simulink library "Library_Betriebsstrategie"  (R2018b)
settings: Solver=VariableStepAuto  StartTime=0.0  StopTime=10.0  RelTol=1e-3  EnableMultiTasking=on
undefined symbols (not defined in the file): akt_eUELG_HA, akt_eUELG_VA, akt_keinMVS_HA, akt_keinMVS_VA, akt_LSD_HA, akt_LSD_VA, akt_mUELG_HA, akt_mUELG_VA, akt_OD_HA, akt_OD_VA, DiscIntNeverNeededParam, magnitude, mu_road, mu_road_LF, mu_road_LR, mu_road_RF, mu_road_RR, par_MDT, par_VEH, stepsize
libraries: simulink x13
(part 6 of 6)

== matlab function Library_Betriebsstrategie/Momentverteilung_LR2/Radmomentenaufteilung/Optimierung rechts/Optimierung rechts ==
  data: M_wheel_right input; omega_RF input; omega_RR input; eta_RF input; eta_RR input; C output; D output; E output; v_slip_RF input; v_slip_RR input; gammaR output; min_P_loss output; Fz_RF input; Fz_RR input; Fy_RF input; Fy_RR input; r input
function [C, D, E, gammaR, min_P_loss] = fcn(M_wheel_right, omega_RF, omega_RR, eta_RF, eta_RR, v_slip_RF, v_slip_RR, Fz_RF, Fz_RR, Fy_RF, Fy_RR, r)

%% Diskrete Variable x (1 Prozent Schritte für Radmomentverteilung) und Initialisierung
step = 0.01;
x = [0:step:1];
n = 1/step + 1;
Einser = ones(1,n);
K_loss = 1;
K_slip = 1;
K_traction = 10;

%% Leistungsverluste in Abhängigkeit vom Antreiben oder Rekuperieren
if M_wheel_right >= 0 %vorne
    P_loss_f = ((Einser ./ eta_RF - 1)*omega_RF*M_wheel_right) .* x;
else
    P_loss_f = ((1 - eta_RF)*omega_RF*M_wheel_right) .* x;
end

if M_wheel_right >= 0 %hinten
    P_loss_r = ((Einser ./ eta_RR - 1)*omega_RR*M_wheel_right) .* (1-x);
else
    P_loss_r = ((1 - eta_RR)*omega_RR*M_wheel_right) .* (1-x);
end

%% Leistungsverluste in Abhängigkeit des Radschlupfes (also wird Traktion auch mit berücksichtigt)
P_slip_f = 5* abs(v_slip_RF * M_wheel_right/r) .* x;

P_slip_r = 5* abs(v_slip_RR * M_wheel_right/r) .* (1-x);

%% Ausnutzung des Kraftführungspotentials
mueT_RF = ((((M_wheel_right/r).*x).^2 + Fy_RF^2) ./ Fz_RF).^0.5;
mueT_RR = ((((M_wheel_right/r).*(1-x)).^2 + Fy_RR^2) ./ Fz_RR).^0.5;

%% Minimum der diskreten Leistungsverluste
P_loss = K_loss*(P_loss_f + P_loss_r) + K_slip*(P_slip_f + P_slip_r) + K_traction*(mueT_RF + mueT_RR);
[A, B] = min(P_loss);

%% Wertezuweisung
gammaR = step*B - step;
min_P_loss = A;

%% Analyse der Gewichtung bzw der Anteile an der Minimierungsfunktion
P_slip_rechts = K_slip*(P_slip_f + P_slip_r);
P_loss_rechts = K_loss*(P_loss_f + P_loss_r);
P_traction_rechts = K_traction*(mueT_RF + mueT_RR);
[C] = min(P_slip_rechts);
[D] = min(P_loss_rechts);
[E] = min(P_traction_rechts);

== matlab function Library_Betriebsstrategie/Momentverteilung_LR2/Limitierungen gesamt (mit MVS Limits)/Subsystem/MATLAB Function ==
  data: L1 input; Delta_T_f output; L2 input; L3 input; L4 input; L5 input; a_f input; a_r input; Delta_T_r output
function [Delta_T_f, Delta_T_r]  = fcn(L1, L2, L3, L4, L5, a_f, a_r)

%% Initialisierung
Delta_T_f=0;
Delta_T_r=0;

%% Zuweisung der maximalen TV Momente anhand der Antriebsstrangtopologie
if a_f == 3
    Delta_T_f=L5;
elseif a_f == 4
    Delta_T_f=L1;
elseif a_f == 5;
    Delta_T_f=L2;
end

if a_r == 3
    Delta_T_r=L5;
elseif a_r == 4
    Delta_T_r=L1;
elseif a_r == 5;
    Delta_T_r=L2;
end

%% Nomenklatur der Aktuatoren a_r und a_f
    % 1 = nur Elektromaschinen an der Achse
    % 2 = Offenes Differential an der Achse
    % 3 = Limited Slip Differential an der Achse
    % 4 = Elektrisches Überlagerungsgetriebe an der Achse
    % 5 = Mechanisches Überlagerungsgetriebe an der Achse

== matlab function Library_Betriebsstrategie/Momentenverteilung_Lagrange1/Limitierungen gesamt (mit MVS Limits)/Aktuatoren und Delta TV/Zuweisung Aktuatoren ==
  data: A1 input; A2 input; A3 input; A4 input; A5 input; a_f output; a_r output; A6 input; A7 input; A8 input; A9 input; A10 input
function [a_f, a_r]  = fcn(A1, A2, A3, A4, A5, A6, A7, A8, A9, A10)

%% Initialisierung
a_f=1;
a_r=1;

%% Zuweisung der Aktuatoren
% vorne
if A1 == 1
    a_f = 2;
elseif A2 == 1
    a_f = 3;
elseif A3 == 1
    a_f = 5;
elseif A4 == 1
    a_f = 4;
elseif A5 == 1
    a_f = 1;
end

% hinten
if A6 == 1
    a_r = 2;
elseif A7 == 1
    a_r = 3;
elseif A8 == 1
    a_r = 5;
elseif A9 == 1
    a_r = 4;
elseif A10 == 1
    a_r = 1;
end

%% Nomenklatur der Aktuatoren a_r und a_f
    % 1 = nur Elektromaschinen an der Achse
    % 2 = Offenes Differential an der Achse
    % 3 = Limited Slip Differential an der Achse
    % 4 = Elektrisches Überlagerungsgetriebe an der Achse
    % 5 = Mechanisches Überlagerungsgetriebe an der Achse

== matlab function Library_Betriebsstrategie/Momentenverteilung_Lagrange1/Limitierungen gesamt (mit MVS Limits)/Aktuatoren und Delta TV/TV Moment pro Achse ==
  data: L1 input; Delta_T_f output; L2 input; L3 input; L4 input; L5 input; a_f input; a_r input; Delta_T_r output
function [Delta_T_f, Delta_T_r]  = fcn(L1, L2, L3, L4, L5, a_f, a_r)

%% Initialisierung
Delta_T_f=0;
Delta_T_r=0;

%% Zuweisung der maximalen TV Momente anhand der Antriebsstrangtopologie
if a_f == 3
    Delta_T_f=L5;
elseif a_f == 4
    Delta_T_f=L1;
elseif a_f == 5;
    Delta_T_f=L2;
end

if a_r == 3
    Delta_T_r=L5;
elseif a_r == 4
    Delta_T_r=L1;
elseif a_r == 5;
    Delta_T_r=L2;
end

%% Nomenklatur der Aktuatoren a_r und a_f
    % 1 = nur Elektromaschinen an der Achse
    % 2 = Offenes Differential an der Achse
    % 3 = Limited Slip Differential an der Achse
    % 4 = Elektrisches Überlagerungsgetriebe an der Achse
    % 5 = Mechanisches Überlagerungsgetriebe an der Achse

== matlab function Library_Betriebsstrategie/Momentenverteilung_Lagrange1/Limitierungen gesamt (mit MVS Limits)/Limits Zusammenführung ==
  data: FxlimRF input; FxlimLF input; FxlimRR input; Fx_LF_ub output; Fx_LF_lb output; Fx_RF_ub output; Fx_RF_lb output; Fx_LR_ub output; Fx_LR_lb output; Fx_RR_ub output; Fx_RR_lb output; FxlimLR input; M_RF_ub input; M_RF_lb input; M_LF_ub input; M_LF_lb input; M_RR_ub input; M_RR_lb input; M_LR_ub input; M_LR_lb input; M_F_lb input; M_F_ub input; M_R_lb input; M_R_ub input; DELTA_T_f input; DELTA_T_r input; a_f input; a_r input; r input
function [Fx_LF_ub, Fx_LF_lb, Fx_RF_ub, Fx_RF_lb, Fx_LR_ub, Fx_LR_lb, Fx_RR_ub, Fx_RR_lb] = fcn(FxlimRF, FxlimLF, FxlimRR, FxlimLR, M_RF_ub, M_RF_lb, M_LF_ub, M_LF_lb, M_RR_ub, M_RR_lb, M_LR_ub, M_LR_lb, M_F_lb, M_F_ub, M_R_lb, M_R_ub,DELTA_T_f, DELTA_T_r,a_f, a_r, r)

%% Initialisierung der Limitationen auf die Reifen-Limits
Fx_LF_ub = FxlimLF;
Fx_RF_ub = FxlimRF;
Fx_LF_lb = (-1*FxlimLF);
Fx_RF_lb = (-1*FxlimRF);

Fx_LR_ub = FxlimLR;
Fx_RR_ub = FxlimRR;
Fx_LR_lb = (-1*FxlimLR);
Fx_RR_lb = (-1*FxlimRR);
    
%% Nomenklatur der Aktuatoren a_r und a_f
    % 1 = nur Elektromaschinen an der Achse
    % 2 = Offenes Differential an der Achse
    % 3 = Limited Slip Differential an der Achse
    % 4 = Elektrisches Überlagerungsgetriebe an der Achse
    % 5 = Mechanisches Überlagerungsgetriebe an der Achse
 
    
%% Nur Elektromotoren: Limit ist Minimum/Maximum aus Reifenlimit und Limit der EM
if a_f == 1
    Fx_LF_ub = min(FxlimLF,(M_LF_ub/r));
    Fx_RF_ub = min(FxlimRF,(M_RF_ub/r));
    Fx_LF_lb = max((-1*FxlimLF),(M_LF_lb/r));
    Fx_RF_lb = max((-1*FxlimRF),(M_RF_lb/r));
end

if a_r == 1
    Fx_LR_ub = min(FxlimLR,(M_LR_ub/r));
    Fx_RR_ub = min(FxlimRR,(M_RR_ub/r));
    Fx_LR_lb = max((-1*FxlimLR),(M_LR_lb/r));
    Fx_RR_lb = max((-1*FxlimRR),(M_RR_lb/r));
end

%% Offenes Differential: Limit ist Minimum/Maximum aus Reifenlimit und genau der Hälfte des max. Moments der achszentralen EM
if a_f == 2
    Fx_LF_ub = min(FxlimLF,(0.5*M_F_ub/r));
    Fx_RF_ub = min(FxlimRF,(0.5*M_F_ub/r));
    Fx_LF_lb = max((-1*FxlimLF),(0.5*M_F_lb/r));
    Fx_RF_lb = max((-1*FxlimRF),(0.5*M_F_lb/r));
end

if a_r == 2
    Fx_LR_ub = min(FxlimLR,(0.5*M_R_ub/r));
    Fx_RR_ub = min(FxlimRR,(0.5*M_R_ub/r));
    Fx_LR_lb = max((-1*FxlimLR),(0.5*M_R_lb/r));
    Fx_RR_lb = max((-1*FxlimRR),(0.5*M_R_lb/r));
end

%% Limited Slip Differential %% Elektrisches Überlagerungsgetriebe %% Mechanisches Überlagerungsgetriebe
if a_f >= 3 
    Fx_LF_ub = min(FxlimLF,(0.5*M_F_ub/r + 0.5*DELTA_T_f/r));
    Fx_RF_ub = min(FxlimRF,(0.5*M_F_ub/r + 0.5*DELTA_T_f/r));
    Fx_LF_lb = max((-1*FxlimLF),(0.5*M_F_lb/r - 0.5*DELTA_T_f/r));
    Fx_RF_lb = max((-1*FxlimRF),(0.5*M_F_lb/r - 0.5*DELTA_T_f/r));
end

if a_r >= 3
    Fx_LR_ub = min(FxlimLR,(0.5*M_R_ub/r + 0.5*DELTA_T_r/r));
    Fx_RR_ub = min(FxlimRR,(0.5*M_R_ub/r + 0.5*DELTA_T_r/r));
    Fx_LR_lb = max((-1*FxlimLR),(0.5*M_R_lb/r - 0.5*DELTA_T_r/r));
    Fx_RR_lb = max((-1*FxlimRR),(0.5*M_R_lb/r - 0.5*DELTA_T_r/r));
end

== matlab function Library_Betriebsstrategie/Momentenverteilung_Lagrange1/Radmomentenaufteilung/Limits berücksichtigen ==
  data: Fx_RF output; Fx_LF output; Fx_RR output; Fx_LF_ub input; Fx_LF_lb input; Fx_RF_ub input; Fx_RF_lb input; Fx_LR_ub input; Fx_LR_lb input; Fx_RR_ub input; Fx_RR_lb input; a_f input; a_r input; Fx_LR output; X_FL input; X_FR input; X_RL input; X_RR input
function [Fx_RF, Fx_LF, Fx_RR, Fx_LR] = fcn(Fx_LF_ub, Fx_LF_lb, Fx_RF_ub, Fx_RF_lb, Fx_LR_ub, Fx_LR_lb, Fx_RR_ub, Fx_RR_lb,a_f, a_r, X_FL, X_FR, X_RL, X_RR)

%% Initialisierung
Fx_RF = X_FR;
Fx_LF = X_FL;
Fx_RR = X_RR;
Fx_LR = X_RL;
    
%% Nomenklatur der Aktuatoren a_r und a_f
    % 1 = nur Elektromaschinen an der Achse
    % 2 = Offenes Differential an der Achse
    % 3 = Limited Slip Differential an der Achse
    % 4 = Elektrisches Überlagerungsgetriebe an der Achse
    % 5 = Mechanisches Überlagerungsgetriebe an der Achse
 
%% Algorithmus

    F_f= Fx_RF+Fx_LF;
    F_r= Fx_RR+Fx_LR;
  
  % Nur Elektromotoren:
  % Es werden radindividuell die Grenzen eingehalten. Die Differenzkräfte
  % werden zur späteren Verwendung gespeichert.
if a_f ==1
    if Fx_LF > Fx_LF_ub
        dFx_LF = Fx_LF-Fx_LF_ub;
        Fx_LF = Fx_LF_ub;
    end
    if Fx_RF > Fx_RF_ub
        dFx_RF = Fx_RF-Fx_RF_ub;
        Fx_RF = Fx_RF_ub;
    end
    if Fx_LF < Fx_LF_lb
        dFx_LF = Fx_LF-Fx_LF_lb;
        Fx_LF = Fx_LF_lb;
    end
    if Fx_RF < Fx_RF_lb
        dFx_RF = Fx_RF-Fx_RF_lb;
        Fx_RF = Fx_RF_lb;
    end
end

if a_r ==1
    if Fx_LR > Fx_LR_ub
        dFx_LR = Fx_LR-Fx_LR_ub;
        Fx_LR = Fx_LR_ub;
    end
    if Fx_RR > Fx_RR_ub
        dFx_RR = Fx_RR-Fx_RR_ub;
        Fx_RR = Fx_RR_ub;
    end
    if Fx_LR < Fx_LR_lb
        dFx_LR = Fx_LR-Fx_LR_lb;
        Fx_LR = Fx_LR_lb;
    end
    if Fx_RR < Fx_RR_lb
        dFx_RR = Fx_RR-Fx_RR_lb;
        Fx_RR = Fx_RR_lb;
    end
end

  % Offenes Differential:
  % ALSO keine TV Funktion der Achse.
  % Jedes Rad erhält die Hälfte der Gesamtachskraft.
  % Anschließend wird diese Kraft auf das Minimum der einzelnen Limits
  % gedeckelt.
  
if a_f ==2
    Fx_LF = F_f/2;
    Fx_RF = F_f/2;
    if Fx_LF > Fx_LF_ub || Fx_RF > Fx_RF_ub
        Fx_LF = min(Fx_LF_ub,Fx_RF_ub);
        Fx_RF = Fx_LF;
    end
    if Fx_LF < Fx_LF_lb || Fx_RF < Fx_RF_lb
        Fx_LF = max(Fx_LF_lb,Fx_RF_lb);
        Fx_RF = Fx_LF;
    end
end

if a_r ==2
    Fx_LR = F_r/2;
    Fx_RR = F_r/2;
    if Fx_LR > Fx_LR_ub || Fx_RR > Fx_RR_ub
        Fx_LR = min(Fx_LR_ub,Fx_RR_ub);
        Fx_RR = Fx_LR;
    end
    if Fx_LR < Fx_LR_lb || Fx_RR < Fx_RR_lb
        Fx_LR = max(Fx_LR_lb,Fx_RR_lb);
        Fx_RR = Fx_LR;
    end
end
    
%% Limited Slip Differential %% Elektrisches Überlagerungsgetriebe %% Mechanisches Überlagerungsgetriebe
if a_f >=3
    if Fx_LF > Fx_LF_ub
        dFx_LF = Fx_LF-Fx_LF_ub;
        Fx_LF = Fx_LF_ub;
    end
    if Fx_RF > Fx_RF_ub
        dFx_RF = Fx_RF-Fx_RF_ub;
        Fx_RF = Fx_RF_ub;
    end
    if Fx_LF < Fx_LF_lb
        dFx_LF = Fx_LF-Fx_LF_lb;
        Fx_LF = Fx_LF_lb;
    end
    if Fx_RF < Fx_RF_lb
        dFx_RF = Fx_RF-Fx_RF_lb;
        Fx_RF = Fx_RF_lb;
    end
end

if a_r >=3
    if Fx_LR > Fx_LR_ub
        dFx_LR = Fx_LR-Fx_LR_ub;
        Fx_LR = Fx_LR_ub;
    end
    if Fx_RR > Fx_RR_ub
        dFx_RR = Fx_RR-Fx_RR_ub;
        Fx_RR = Fx_RR_ub;
    end
    if Fx_LR < Fx_LR_lb
        dFx_LR = Fx_LR-Fx_LR_lb;
        Fx_LR = Fx_LR_lb;
    end
    if Fx_RR < Fx_RR_lb
        dFx_RR = Fx_RR-Fx_RR_lb;
        Fx_RR = Fx_RR_lb;
    end
end
    
%% Korrektur des TV Moments %% Korrektur des Gesamtmoments

== matlab function Library_Betriebsstrategie/Momentenverteilung_Lagrange1/Radmomentenaufteilung/Optimierung mit Lagrange Multiplikator Methode ==
  data: a_f input; a_r input; vslip_FL input; vslip_FR input; vslip_RL input; vslip_RR input; tF input; tR input; lf input; lr input; delta input; X_req input; Mz input; X_FL output; X_FR output; X_RL output; X_RR output; Z_FL input; Z_FR input; Z_RL input; Z_RR input; X_FL1 input; X_FR1 input; X_RL1 input; X_RR1 input
function [X_FL, X_FR, X_RL, X_RR] = fcn(a_f, a_r, vslip_FL, vslip_FR, vslip_RL, vslip_RR,tF, tR, lf, lr, delta, X_req, Mz, Z_FL, Z_FR, Z_RL, Z_RR, X_FL1, X_FR1, X_RL1, X_RR1)

%% Auswahl der Antriebsstrantopologie
a=1;
b=1;

if a_f ==2
    a=0;
end
if a_r ==2
    b=0;
end

if a_f ==2 && a_r==2
    a=1;
    b=1;
end

% TV vorne und hinten möglich a=1 und b=1
% TV nur vorne möglich a=1
% TV nur hinten möglich b=1
% kein TV möglich a=0 und b=0

%% Matrix für die Randbedingungen ( Gesamtmoment und TV Moment)
B0 = [cos(delta) cos(delta) 1 1; a*((-tF/2)*cos(delta)+lf*sin(delta)) a*((tF/2)*cos(delta)+lf*sin(delta)) b*(-tR/2) b*(tR/2)];
y0 = [X_req; Mz];

%% Algorithmus
    %% Initialbedingungen
i=0;    
B=B0;
y=y0;
     
    %% Verhindern abgehobener Räder
if Z_FL < 1
    Z_FL = 1;
    x_FL_max = 0;
end

if Z_FR < 1
    Z_FR = 1;
    x_FR_max = 0;
end

if Z_RL < 1
    Z_RL = 1;
    x_RL_max = 0;
end

if Z_RR < 1
    Z_RR = 1;
    x_RR_max = 0;
end

%% Matrizen für die Mimimierung
W1 = [1/Z_FL+abs(vslip_FL) 0 0 0; 0 1/Z_FR+abs(vslip_FR) 0 0; 0 0 1/Z_RL+abs(vslip_RL) 0; 0 0 0 1/Z_RR+abs(vslip_RR)];
W2 = 0.01 * eye(4);
Wquad = W1^2 + W2^2;
X_alt = [X_FL1; X_FR1; X_RL1; X_RR1];

%% Minimierungsargument
% min ||W1*x||^2 + ||W2*(x-x0)||^2
%   ||W1*x||^2 + ||W2*(x-x0)||^2 = xt*W1^2*x + (x-x0)t*W2^2*(x-x0)
%   = xt*(W1^2+W2^2)*x - 2*x*W2^2*x0 + x0*W2^2*x0
%   = xt*W^2*x - 2*x*W2^2*x0 + Konstante
%   mit W^2 = W1^2 + W2^2


%% Berechnung von Xij
G = (Wquad^(-1))*(B')*(B*(Wquad^(-1))*(B'))^(-1);
X = G*y + (eye(4)-G*B)*(Wquad^(-1))*(W2^2)*X_alt;


%% Ausgabewerte berechnen
X_FL = X(1);
X_FR = X(2);
X_RL = X(3);
X_RR = X(4);

%% Limits berücksichtigen
if a==0
    X_F = X_FL + X_FR;
    X_FL = X_F/2;
    X_FR = X_F/2;
end

if b==0
    X_R = X_RL + X_RR;
    X_RL = X_R/2;
    X_RR = X_R/2;
end

if a_f ==2 && a_r==2
    X_F = X_FL + X_FR;
    X_FL = X_F/2;
    X_FR = X_F/2;
    X_R = X_RL + X_RR;
    X_RL = X_R/2;
    X_RR = X_R/2;
end

== matlab function Library_Betriebsstrategie/Schaltstrategie/Schaltlogik ==
  data: delta_n_LF input; delta_n_RF input; delta_n_LR input; delta_n_RR input; delta_n_F input; delta_n_R input; delta_m_LF input; delta_m_RF input; delta_m_LR input; delta_m_RR input; delta_m_F input; delta_m_R input; idx_LF_eff input; idx_RF_eff input; idx_LR_eff input; idx_RR_eff input; idx_F_eff input; idx_R_eff input; i_LF output; i_RF output; i_LR output; i_RR output; i_F output; iv_LF input; iv_RF input; iv_LR input; iv_RR input; iv_F input; iv_R input; i_R output; idx_LF output; idx_RF output; idx_LR output; idx_RR output; idx_F output; idx_R output; idx_LF_alt input; idx_RF_alt input; idx_LR_alt input; idx_RR_alt input; idx_F_alt input; idx_R_alt input
function [i_LF, i_RF, i_LR, i_RR, i_F, i_R, idx_LF, idx_RF, idx_LR, idx_RR, idx_F, idx_R] = fcn(delta_n_LF, delta_n_RF, delta_n_LR, delta_n_RR, delta_n_F, delta_n_R, delta_m_LF, delta_m_RF, delta_m_LR, delta_m_RR, delta_m_F, delta_m_R, idx_LF_eff, idx_RF_eff, idx_LR_eff, idx_RR_eff, idx_F_eff, idx_R_eff, iv_LF, iv_RF, iv_LR, iv_RR, iv_F, iv_R, idx_LF_alt, idx_RF_alt, idx_LR_alt, idx_RR_alt, idx_F_alt, idx_R_alt)

%% Anzahl der möglichen Gänge
[A,max_LF]=size(iv_LF);
[A,max_RF]=size(iv_RF);
[A,max_LR]=size(iv_LR);
[A,max_RR]=size(iv_RR);
[A,max_F]=size(iv_F);
[A,max_R]=size(iv_R);

flag_LF=0;
flag_RF=0;
flag_LR=0;
flag_RR=0;
flag_F=0;
flag_R=0;


%% LF
idx_LF=idx_LF_alt;

if delta_n_LF<100 && idx_LF_alt<max_LF
    idx_LF=idx_LF_alt+1;
    flag_LF=1;
end

if delta_m_LF<1 && idx_LF_alt>1 && flag_LF==0
    idx_LF=idx_LF_alt-1;
    flag_LF=1;
end
    
if flag_LF==0
    idx_LF=idx_LF_eff;
end

i_LF=iv_LF(idx_LF);

%% RF
idx_RF=idx_RF_alt;

if delta_n_RF<100 && idx_RF_alt<max_RF
    idx_RF=idx_RF_alt+1;
    flag_RF=1;
end

if delta_m_RF<1 && idx_RF_alt>1 && flag_RF==0
    idx_RF=idx_RF_alt-1;
    flag_RF=1;
end
    
if flag_RF==0
    idx_RF=idx_RF_eff;
end

i_RF=iv_RF(idx_RF);

%% LR
idx_LR=idx_LR_alt;

if delta_n_LR<100 && idx_LR_alt<max_LR
    idx_LR=idx_LR_alt+1;
    flag_LR=1;
end

if delta_m_LR<1 && idx_LR_alt>1 && flag_LR==0
    idx_LR=idx_LR_alt-1;
    flag_LR=1;
end
    
if flag_LR==0
    idx_LR=idx_LR_eff;
end

i_LR=iv_LR(idx_LR);

%% RR
idx_RR=idx_RR_alt;

if delta_n_RR<100 && idx_RR_alt<max_RR
    idx_RR=idx_RR_alt+1;
    flag_RR=1;
end

if delta_m_RR<1 && idx_RR_alt>1 && flag_RR==0
    idx_RR=idx_RR_alt-1;
    flag_RR=1;
end
    
if flag_RR==0
    idx_RR=idx_RR_eff;
end

i_RR=iv_RR(idx_RR);

%% F
idx_F=idx_F_alt;

if delta_n_F<100 && idx_F_alt<max_F
    idx_F=idx_F_alt+1;
    flag_F=1;
end

if delta_m_F<1 && idx_F_alt>1 && flag_F==0
    idx_F=idx_F_alt-1;
    flag_F=1;
end
    
if flag_F==0
    idx_F=idx_F_eff;
end

i_F=iv_F(idx_F);

%% R
idx_R=idx_R_alt;

if delta_n_R<100 && idx_R_alt<max_R
    idx_R=idx_R_alt+1;
    flag_R=1;
end

if delta_m_R<1 && idx_R_alt>1 && flag_R==0
    idx_R=idx_R_alt-1;
    flag_R=1;
end
    
if flag_R==0
    idx_R=idx_R_eff;
end

i_R=iv_R(idx_R);

== matlab function Library_Betriebsstrategie/Schaltstrategie/effizientester Gang ==
  data: eta_LF input; eta_RF input; eta_LR input; eta_RR input; eta_F input; eta_R input; idx_LF_eff output; idx_RF_eff output; idx_LR_eff output; idx_RR_eff output; idx_F_eff output; idx_R_eff output
function [idx_LF_eff, idx_RF_eff, idx_LR_eff, idx_RR_eff, idx_F_eff, idx_R_eff] = fcn(eta_LF, eta_RF, eta_LR, eta_RR, eta_F, eta_R)

%% effizientester Gang Achszentraler Aufbau
[A,B]=max(eta_F);
idx_F_eff=B;

[A,B]=max(eta_R);
idx_R_eff=B;

%% effizientester Gang Radindividueller Aufbau
[A,B]=max(eta_LF);
idx_LF_eff=B;

[A,B]=max(eta_RF);
idx_RF_eff=B;

[A,B]=max(eta_LR);
idx_LR_eff=B;

[A,B]=max(eta_RR);
idx_RR_eff=B;

== matlab function Library_Betriebsstrategie/Schaltstrategie/n und Motordrehmoment als Vektor (wegen ALLEN Übersetzungen) ==
  data: omega_LF input; n_LF output; m_LF output; omega_RF input; omega_LR input; omega_RR input; M_LF input; M_RF input; M_LR input; M_RR input; i_LF input; i_RF input; i_LR input; i_RR input; i_F input; i_R input; n_RF output; m_RF output; n_LR output; m_LR output; n_RR output; m_RR output; n_F output; m_F output; n_R output; m_R output
function [n_LF,m_LF, n_RF,m_RF, n_LR,m_LR, n_RR,m_RR, n_F,m_F, n_R,m_R] = fcn(omega_LF, omega_RF, omega_LR, omega_RR, M_LF, M_RF, M_LR, M_RR, i_LF, i_RF, i_LR, i_RR, i_F, i_R)

%% Drehzahlen und Momente als Vektoren
% Die Menge an möglichen Übersetzungen liegt als Vektor vor.
% Durch Vektoropertaionen werden Drehzahlen und Momente ebenfalls als
% Vektoren dargestellt. Diese werden im Wirkungsgradkennfeld zu einem
% Vektor an Wirkungsgraden. Von diesen wird der beste ausgewählt.

%% Raddrehzahlen Achszentraler Aufbau
n_F = (omega_LF+omega_RF)*0.5.*i_F;
n_R = (omega_LR+omega_RR)*0.5.*i_R;

%% Raddrehzahlen Radindividueller Aufbau
n_LF = omega_LF.*i_LF;
n_RF = omega_RF.*i_RF;
n_LR = omega_LR.*i_LR;
n_RR = omega_RR.*i_RR;

%% Motormoment Achszentraler Aufbau
m_F=(M_LF+M_RF)./i_F;
m_R=(M_LR+M_RR)./i_R;

%% Motormoment Radindividueller Aufbau
m_LF=M_LF./i_LF;
m_RF=M_RF./i_RF;
m_LR=M_LR./i_LR;
m_RR=M_RR./i_RR;

== matlab function Library_Betriebsstrategie/Schaltstrategie/omega zu n ==
  data: omega_LF input; n_LF output; omega_RF input; omega_LR input; omega_RR input; i_LF input; i_RF input; i_LR input; i_RR input; i_F input; i_R input; n_RF output; n_LR output; n_RR output; n_F output; n_R output
function [n_LF, n_RF, n_LR, n_RR, n_F, n_R] = fcn(omega_LF, omega_RF, omega_LR, omega_RR, i_LF, i_RF, i_LR, i_RR, i_F, i_R)

%% Raddrehzahlen Achszentraler Aufbau
n_F = (omega_LF+omega_RF)*0.5*i_F;
n_R = (omega_LR+omega_RR)*0.5*i_R;

%% Raddrehzahlen Radindividueller Aufbau
n_LF = omega_LF*i_LF;
n_RF = omega_RF*i_RF;
n_LR = omega_LR*i_LR;
n_RR = omega_RR*i_RR;

== matlab function Library_Betriebsstrategie/Momentenverteilung_Lagrange2/Limitierungen gesamt (mit MVS Limits)/Aktuatoren und Delta TV/TV Moment pro Achse ==
  data: L1 input; Delta_T_f output; L2 input; L3 input; L4 input; L5 input; a_f input; a_r input; Delta_T_r output
function [Delta_T_f, Delta_T_r]  = fcn(L1, L2, L3, L4, L5, a_f, a_r)

%% Initialisierung
Delta_T_f=0;
Delta_T_r=0;

%% Zuweisung der maximalen TV Momente anhand der Antriebsstrangtopologie
if a_f == 3
    Delta_T_f=L5;
elseif a_f == 4
    Delta_T_f=L1;
elseif a_f == 5;
    Delta_T_f=L2;
end

if a_r == 3
    Delta_T_r=L5;
elseif a_r == 4
    Delta_T_r=L1;
elseif a_r == 5;
    Delta_T_r=L2;
end

%% Nomenklatur der Aktuatoren a_r und a_f
    % 1 = nur Elektromaschinen an der Achse
    % 2 = Offenes Differential an der Achse
    % 3 = Limited Slip Differential an der Achse
    % 4 = Elektrisches Überlagerungsgetriebe an der Achse
    % 5 = Mechanisches Überlagerungsgetriebe an der Achse

== matlab function Library_Betriebsstrategie/Momentenverteilung_Lagrange2/Limitierungen gesamt (mit MVS Limits)/Aktuatoren und Delta TV/Zuweisung Aktuatoren ==
  data: A1 input; A2 input; A3 input; A4 input; A5 input; a_f output; a_r output; A6 input; A7 input; A8 input; A9 input; A10 input
function [a_f, a_r]  = fcn(A1, A2, A3, A4, A5, A6, A7, A8, A9, A10)

%% Initialisierung
a_f=1;
a_r=1;

%% Zuweisung der Aktuatoren
% vorne
if A1 == 1
    a_f = 2;
elseif A2 == 1
    a_f = 3;
elseif A3 == 1
    a_f = 5;
elseif A4 == 1
    a_f = 4;
elseif A5 == 1
    a_f = 1;
end

% hinten
if A6 == 1
    a_r = 2;
elseif A7 == 1
    a_r = 3;
elseif A8 == 1
    a_r = 5;
elseif A9 == 1
    a_r = 4;
elseif A10 == 1
    a_r = 1;
end

%% Nomenklatur der Aktuatoren a_r und a_f
    % 1 = nur Elektromaschinen an der Achse
    % 2 = Offenes Differential an der Achse
    % 3 = Limited Slip Differential an der Achse
    % 4 = Elektrisches Überlagerungsgetriebe an der Achse
    % 5 = Mechanisches Überlagerungsgetriebe an der Achse

== matlab function Library_Betriebsstrategie/Momentenverteilung_Lagrange2/Limitierungen gesamt (mit MVS Limits)/Limits Zusammenführung ==
  data: FxlimRF input; FxlimLF input; FxlimRR input; Fx_LF_ub output; Fx_LF_lb output; Fx_RF_ub output; Fx_RF_lb output; Fx_LR_ub output; Fx_LR_lb output; Fx_RR_ub output; Fx_RR_lb output; FxlimLR input; M_RF_ub input; M_RF_lb input; M_LF_ub input; M_LF_lb input; M_RR_ub input; M_RR_lb input; M_LR_ub input; M_LR_lb input; M_F_lb input; M_F_ub input; M_R_lb input; M_R_ub input; DELTA_T_f input; DELTA_T_r input; a_f input; a_r input; r input
function [Fx_LF_ub, Fx_LF_lb, Fx_RF_ub, Fx_RF_lb, Fx_LR_ub, Fx_LR_lb, Fx_RR_ub, Fx_RR_lb] = fcn(FxlimRF, FxlimLF, FxlimRR, FxlimLR, M_RF_ub, M_RF_lb, M_LF_ub, M_LF_lb, M_RR_ub, M_RR_lb, M_LR_ub, M_LR_lb, M_F_lb, M_F_ub, M_R_lb, M_R_ub,DELTA_T_f, DELTA_T_r,a_f, a_r, r)

% Reifenverhalten beim Antreiben und Bremsen gleich
Fx_LF_ub = FxlimLF;
Fx_RF_ub = FxlimRF;
Fx_LF_lb = (-1*FxlimLF);
Fx_RF_lb = (-1*FxlimRF);

Fx_LR_ub = FxlimLR;
Fx_RR_ub = FxlimRR;
Fx_LR_lb = (-1*FxlimLR);
Fx_RR_lb = (-1*FxlimRR);

% Notwendig, da die Rekuperationskennfelder aus dem Pesche Tool positive
% Momente ausgeben
M_RF_lb=(-1)*M_RF_lb;
M_LF_lb=(-1)*M_LF_lb;
M_RR_lb=(-1)*M_RR_lb;
M_LR_lb=(-1)*M_LR_lb;
M_F_lb=(-1)*M_F_lb;
M_R_lb=(-1)*M_R_lb;
    
%% Nomenklatur der Aktuatoren a_r und a_f
    % 1 = nur Elektromaschinen an der Achse
    % 2 = Offenes Differential an der Achse
    % 3 = Limited Slip Differential an der Achse
    % 4 = Elektrisches Überlagerungsgetriebe an der Achse
    % 5 = Mechanisches Überlagerungsgetriebe an der Achse
 
    
%% Nur Elektromotoren: Limit ist Minimum/Maximum aus Reifenlimit und Limit der EM
if a_f == 1
    Fx_LF_ub = min(FxlimLF,(M_LF_ub/r));
    Fx_RF_ub = min(FxlimRF,(M_RF_ub/r));
    Fx_LF_lb = max((-1*FxlimLF),(M_LF_lb/r));
    Fx_RF_lb = max((-1*FxlimRF),(M_RF_lb/r));
end

if a_r == 1
    Fx_LR_ub = min(FxlimLR,(M_LR_ub/r));
    Fx_RR_ub = min(FxlimRR,(M_RR_ub/r));
    Fx_LR_lb = max((-1*FxlimLR),(M_LR_lb/r));
    Fx_RR_lb = max((-1*FxlimRR),(M_RR_lb/r));
end

%% Offenes Differential: Limit ist Minimum/Maximum aus Reifenlimit und genau der Hälfte des max. Moments der achszentralen EM
if a_f == 2
    Fx_LF_ub = min(FxlimLF,(0.5*M_F_ub/r));
    Fx_RF_ub = min(FxlimRF,(0.5*M_F_ub/r));
    Fx_LF_lb = max((-1*FxlimLF),(0.5*M_F_lb/r));
    Fx_RF_lb = max((-1*FxlimRF),(0.5*M_F_lb/r));
end

if a_r == 2
    Fx_LR_ub = min(FxlimLR,(0.5*M_R_ub/r));
    Fx_RR_ub = min(FxlimRR,(0.5*M_R_ub/r));
    Fx_LR_lb = max((-1*FxlimLR),(0.5*M_R_lb/r));
    Fx_RR_lb = max((-1*FxlimRR),(0.5*M_R_lb/r));
end

%% Limited Slip Differential %% Elektrisches Überlagerungsgetriebe %% Mechanisches Überlagerungsgetriebe:
if a_f >= 3 
    Fx_LF_ub = min(FxlimLF,(0.5*M_F_ub/r + 0.5*DELTA_T_f/r));
    Fx_RF_ub = min(FxlimRF,(0.5*M_F_ub/r + 0.5*DELTA_T_f/r));
    Fx_LF_lb = max((-1*FxlimLF),(0.5*M_F_lb/r - 0.5*DELTA_T_f/r));
    Fx_RF_lb = max((-1*FxlimRF),(0.5*M_F_lb/r - 0.5*DELTA_T_f/r));
end

if a_r >= 3
    Fx_LR_ub = min(FxlimLR,(0.5*M_R_ub/r + 0.5*DELTA_T_r/r));
    Fx_RR_ub = min(FxlimRR,(0.5*M_R_ub/r + 0.5*DELTA_T_r/r));
    Fx_LR_lb = max((-1*FxlimLR),(0.5*M_R_lb/r - 0.5*DELTA_T_r/r));
    Fx_RR_lb = max((-1*FxlimRR),(0.5*M_R_lb/r - 0.5*DELTA_T_r/r));
end

== matlab function Library_Betriebsstrategie/Momentenverteilung_Lagrange2/Radmomentenaufteilung1/Limits berücksichtigen ==
  data: Fx_RF output; Fx_LF output; Fx_RR output; Fx_LF_ub input; Fx_LF_lb input; Fx_RF_ub input; Fx_RF_lb input; Fx_LR_ub input; Fx_LR_lb input; Fx_RR_ub input; Fx_RR_lb input; a_f input; a_r input; Fx_LR output; X_FL input; X_FR input; X_RL input; X_RR input
function [Fx_RF, Fx_LF, Fx_RR, Fx_LR] = fcn(Fx_LF_ub, Fx_LF_lb, Fx_RF_ub, Fx_RF_lb, Fx_LR_ub, Fx_LR_lb, Fx_RR_ub, Fx_RR_lb,a_f, a_r, X_FL, X_FR, X_RL, X_RR)

%% Initialisierung
Fx_RF = X_FR;
Fx_LF = X_FL;
Fx_RR = X_RR;
Fx_LR = X_RL;
    
%% Nomenklatur der Aktuatoren a_r und a_f
    % 1 = nur Elektromaschinen an der Achse
    % 2 = Offenes Differential an der Achse
    % 3 = Limited Slip Differential an der Achse
    % 4 = Elektrisches Überlagerungsgetriebe an der Achse
    % 5 = Mechanisches Überlagerungsgetriebe an der Achse
 
%% Algorithmus

    F_f= Fx_RF+Fx_LF;
    F_r= Fx_RR+Fx_LR;
  
  % Nur Elektromotoren:
  % Es werden radindividuell die Grenzen eingehalten. Die Differenzkräfte
  % werden zur späteren Verwendung gespeichert.
if a_f ==1
    if Fx_LF > Fx_LF_ub
        dFx_LF = Fx_LF-Fx_LF_ub;
        Fx_LF = Fx_LF_ub;
    end
    if Fx_RF > Fx_RF_ub
        dFx_RF = Fx_RF-Fx_RF_ub;
        Fx_RF = Fx_RF_ub;
    end
    if Fx_LF < Fx_LF_lb
        dFx_LF = Fx_LF-Fx_LF_lb;
        Fx_LF = Fx_LF_lb;
    end
    if Fx_RF < Fx_RF_lb
        dFx_RF = Fx_RF-Fx_RF_lb;
        Fx_RF = Fx_RF_lb;
    end
end

if a_r ==1
    if Fx_LR > Fx_LR_ub
        dFx_LR = Fx_LR-Fx_LR_ub;
        Fx_LR = Fx_LR_ub;
    end
    if Fx_RR > Fx_RR_ub
        dFx_RR = Fx_RR-Fx_RR_ub;
        Fx_RR = Fx_RR_ub;
    end
    if Fx_LR < Fx_LR_lb
        dFx_LR = Fx_LR-Fx_LR_lb;
        Fx_LR = Fx_LR_lb;
    end
    if Fx_RR < Fx_RR_lb
        dFx_RR = Fx_RR-Fx_RR_lb;
        Fx_RR = Fx_RR_lb;
    end
end

  % Offenes Differential:
  % ALSO keine TV Funktion der Achse.
  % Jedes Rad erhält die Hälfte der Gesamtachskraft.
  % Anschließend wird diese Kraft auf das Minimum der einzelnen Limits
  % gedeckelt.

  %Berücksichtigung bereits in Lagrange-Block
  
% if a_f ==2
%     Fx_LF = F_f/2;
%     Fx_RF = F_f/2;
%     if Fx_LF > Fx_LF_ub || Fx_RF > Fx_RF_ub
%         Fx_LF = min(Fx_LF_ub,Fx_RF_ub);
%         Fx_RF = Fx_LF;
%     end
%     if Fx_LF < Fx_LF_lb || Fx_RF < Fx_RF_lb
%         Fx_LF = max(Fx_LF_lb,Fx_RF_lb);
%         Fx_RF = Fx_LF;
%     end
% end
% 
% if a_r ==2
%     Fx_LR = F_r/2;
%     Fx_RR = F_r/2;
%     if Fx_LR > Fx_LR_ub || Fx_RR > Fx_RR_ub
%         Fx_LR = min(Fx_LR_ub,Fx_RR_ub);
%         Fx_RR = Fx_LR;
%     end
%     if Fx_LR < Fx_LR_lb || Fx_RR < Fx_RR_lb
%         Fx_LR = max(Fx_LR_lb,Fx_RR_lb);
%         Fx_RR = Fx_LR;
%     end
% end
    
%% Limited Slip Differential %% Elektrisches Überlagerungsgetriebe %% Mechanisches Überlagerungsgetriebe
if a_f >=3
    if Fx_LF > Fx_LF_ub
        dFx_LF = Fx_LF-Fx_LF_ub;
        Fx_LF = Fx_LF_ub;
    end
    if Fx_RF > Fx_RF_ub
        dFx_RF = Fx_RF-Fx_RF_ub;
        Fx_RF = Fx_RF_ub;
    end
    if Fx_LF < Fx_LF_lb
        dFx_LF = Fx_LF-Fx_LF_lb;
        Fx_LF = Fx_LF_lb;
    end
    if Fx_RF < Fx_RF_lb
        dFx_RF = Fx_RF-Fx_RF_lb;
        Fx_RF = Fx_RF_lb;
    end
end

if a_r >=3
    if Fx_LR > Fx_LR_ub
        dFx_LR = Fx_LR-Fx_LR_ub;
        Fx_LR = Fx_LR_ub;
    end
    if Fx_RR > Fx_RR_ub
        dFx_RR = Fx_RR-Fx_RR_ub;
        Fx_RR = Fx_RR_ub;
    end
    if Fx_LR < Fx_LR_lb
        dFx_LR = Fx_LR-Fx_LR_lb;
        Fx_LR = Fx_LR_lb;
    end
    if Fx_RR < Fx_RR_lb
        dFx_RR = Fx_RR-Fx_RR_lb;
        Fx_RR = Fx_RR_lb;
    end
end
    
%% Korrektur des TV Moments %% Korrektur des Gesamtmoments

== matlab function Library_Betriebsstrategie/Momentenverteilung_Lagrange2/Radmomentenaufteilung1/Optimierung mit Lagrange Multiplikator Methode ==
  data: a_f input; a_r input; vslip_FL input; vslip_FR input; vslip_RL input; vslip_RR input; tF input; tR input; lf input; lr input; delta input; X_req input; Mz input; X_FL output; X_FR output; X_RL output; X_RR output; Z_FL input; Z_FR input; Z_RL input; Z_RR input; X_FL1 input; X_FR1 input; X_RL1 input; X_RR1 input
function [X_FL, X_FR, X_RL, X_RR] = fcn(a_f, a_r, vslip_FL, vslip_FR, vslip_RL, vslip_RR,tF, tR, lf, lr, delta, X_req, Mz, Z_FL, Z_FR, Z_RL, Z_RR, X_FL1, X_FR1, X_RL1, X_RR1)

%% Auswahl der Antriebsstrantopologie
a=1;
b=1;

if a_f ==2
    a=0;
end
if a_r ==2
    b=0;
end

if a_f ==2 && a_r==2
    a=1;
    b=1;
end

% TV vorne und hinten möglich a=1 und b=1
% TV nur vorne möglich a=1
% TV nur hinten möglich b=1
% kein TV möglich a=1 und b=1 und anschließend gleichmäßig aufteilen

%% Matrix für die Randbedingungen ( Gesamtmoment und TV Moment)
% B0 = [cos(delta) cos(delta) 1 1; a*((-tF/2)*cos(delta)+lf*sin(delta)) a*((tF/2)*cos(delta)+lf*sin(delta)) b*(-tR/2) b*(tR/2)];
% Die Berücksichtigung der Lenkwinkel für die Formel des Gesamtmoments und des Giermomenmts ist exakt, wird
% aber hier erstmal auskommentiert, da ein instabiler Fahrerregler
% vorliegt. Sobald der Fahrerregler komplett stabil ist, kann die obere
% Matrix für B0 verwendet werden.
B0 = [1 1 1 1; a*(-tF/2) a*(tF/2) b*(-tR/2) b*(tR/2)];
y0 = [X_req; Mz];

%% Algorithmus
    %% Initialbedingungen
i=0;    
B=B0;
y=y0;
     
    %% Verhindern abgehobener Räder
if Z_FL < 1
    Z_FL = 1;
    x_FL_max = 0;
end

if Z_FR < 1
    Z_FR = 1;
    x_FR_max = 0;
end

if Z_RL < 1
    Z_RL = 1;
    x_RL_max = 0;
end

if Z_RR < 1
    Z_RR = 1;
    x_RR_max = 0;
end

%% Matrizen für die Mimimierung
W1 = [1/Z_FL 0 0 0; 0 1/Z_FR 0 0; 0 0 1/Z_RL 0; 0 0 0 1/Z_RR];
% W1 = [1/Z_FL+abs(vslip_FL) 0 0 0; 0 1/Z_FR+abs(vslip_FR) 0 0; 0 0 1/Z_RL+abs(vslip_RL) 0; 0 0 0 1/Z_RR+abs(vslip_RR)];
W2 = 0.01 * eye(4);
Wquad = W1^2 + W2^2;
X_alt = [X_FL1; X_FR1; X_RL1; X_RR1];

%% Minimierungsargument
% min ||W1*x||^2 + ||W2*(x-x0)||^2
%   ||W1*x||^2 + ||W2*(x-x0)||^2 = xt*W1^2*x + (x-x0)t*W2^2*(x-x0)
%   = xt*(W1^2+W2^2)*x - 2*x*W2^2*x0 + x0*W2^2*x0
%   = xt*W^2*x - 2*x*W2^2*x0 + Konstante
%   mit W^2 = W1^2 + W2^2

%% Berechnung von Xij
G = (Wquad^(-1))*(B')*(B*(Wquad^(-1))*(B'))^(-1);
X = G*y + (eye(4)-G*B)*(Wquad^(-1))*(W2^2)*X_alt;


%% Ausgabewerte berechnen
X_FL = X(1);
X_FR = X(2);
X_RL = X(3);
X_RR = X(4);

%% Limits berücksichtigen
if a==0
    X_F = X_FL + X_FR;
    X_FL = X_F/2;
    X_FR = X_F/2;
end

if b==0
    X_R = X_RL + X_RR;
    X_RL = X_R/2;
    X_RR = X_R/2;
end

if a_f ==2 && a_r==2
    X_F = X_FL + X_FR;
    X_FL = X_F/2;
    X_FR = X_F/2;
    X_R = X_RL + X_RR;
    X_RL = X_R/2;
    X_RR = X_R/2;
end

== matlab function Library_Betriebsstrategie/Optimierung ==
  data: P_achs input; P_opt output; ind output; M_target input
function [P_opt, ind]= fcn(P_achs, M_target)

if M_target>0
    [P_opt, ind] = min(P_achs(:));
else
    [P_opt, ind] = max(P_achs(:));
end

end
